simulink model "Aufgabe2_10"  (R2024b)
settings: Solver=ode4  StartTime=0.0  StopTime=200  FixedStep=0.01  RelTol=1e-3
values from neighbouring files (symbols this model uses):
  g = 9.807    [start.m]
undefined symbols (not defined in the file or in its folder): ft, INI, m, s
libraries: aerolibconvert2 x5, aerolibasang x4, slpidlib x3, aerolibanimutils x2, aerolibfltsims x2, simulink_extras x1, aerolibatmos2 x1, shared6dof x1
settings Model: Creator=annaf  LastModifiedBy=FrederikRittervonBae

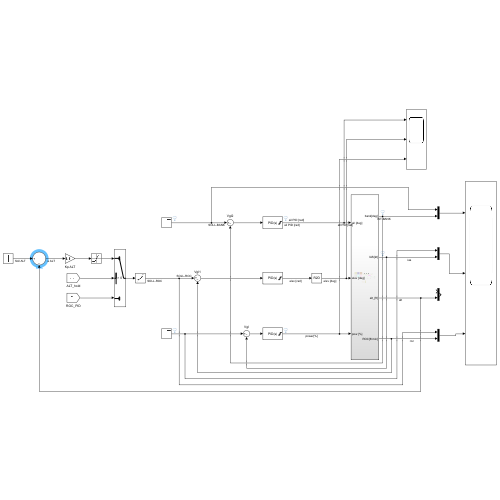
[thumbnail: Simulink's stored preview of the top-level diagram]
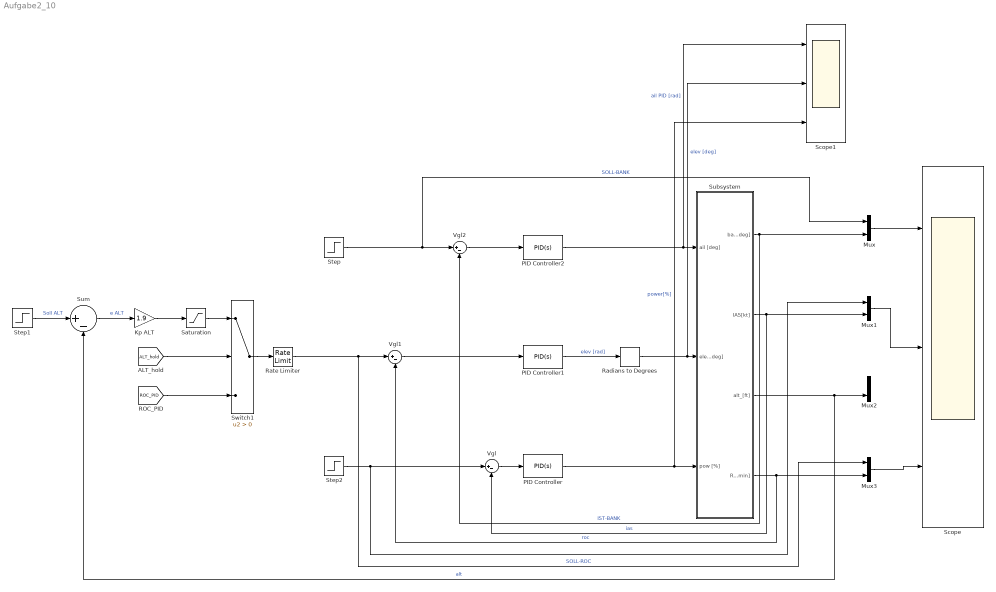
== system Aufgabe2_10 ==
  Kp ALT : Gain  Gain=1.9
  Mux{,1..3} (4 alike) : Mux  Inputs=2
  PID Controller : slpidlib/PID Controller  Controller=PID  Form=Parallel  TimeDomain=Continuous-time  UseExternalTs=off  SampleTime=-1  IntegratorMethod=Forward Euler  FilterMethod=Forward Euler  ControllerParametersSource=internal  P=68.6  I=5.4  UseKiTs=off  D=0.6  UseExternalDerivativeSource=off  N=100  UseFilter=on  TunerSelectOption=Transfer Function Based (PID Tuner App)  InitialConditionSource=internal  InitialConditionForIntegrator=0  InitialConditionForFilter=0  DifferentiatorICPrevScaledInput=0  ExternalReset=none  TrackingMode=off  Kt=1  LimitOutput=on  SatLimitsSource=internal  UpperSaturationLimit=100  LowerSaturationLimit=0  LinearizeAsGain=on  AntiWindupMode=clamping  Kb=1  LimitIntegrator=off  UpperIntegratorSaturationLimit=inf  LowerIntegratorSaturationLimit=-inf  POutMin=[]  POutMax=[]  IOutMin=[]  IOutMax=[]  DOutMin=[]  DOutMax=[]  NOutMin=[]  NOutMax=[]  SumOutMin=[]  SumOutMax=[]  SaturationOutMin=[]  SaturationOutMax=[]  PParamMin=[]  PParamMax=[]  IParamMin=[]  IParamMax=[]  DParamMin=[]  DParamMax=[]  NParamMin=[]  NParamMax=[]  KbParamMin=[]  KbParamMax=[]  KtParamMin=[]  KtParamMax=[]  KbOutMin=[]  KbOutMax=[]  KtOutMin=[]  KtOutMax=[]  IntegratorOutMin=[]  IntegratorOutMax=[]  FilterOutMin=[]  FilterOutMax=[]  SumI1OutMin=[]  SumI1OutMax=[]  SumI2OutMin=[]  SumI2OutMax=[]  SumI3OutMin=[]  SumI3OutMax=[]  SumI4OutMin=[]  SumI4OutMax=[]  SumDOutMin=[]  SumDOutMax=[]  DifferentiatorOutMin=[]  DifferentiatorOutMax=[]  FilterDiffOutCoefMin=[]  FilterDiffOutCoefMax=[]  ReciprocalOutMin=[]  ReciprocalOutMax=[]  SumDenOutMin=[]  SumDenOutMax=[]  SumNumOutMin=[]  SumNumOutMax=[]  DivideOutMin=[]  DivideOutMax=[]  UdiffTsProdOutMin=[]  UdiffTsProdOutMax=[]  NTsProdOutMin=[]  NTsProdOutMax=[]  UintegralTsProdOutMin=[]  UintegralTsProdOutMax=[]  UngainTsProdOutMin=[]  UngainTsProdOutMax=[]  ClampingZeroOutDataTypeStr=Inherit: Inherit via back propagation  ClampingZeroOutMin=[]  ClampingZeroOutMax=[]  FilterDenConstantOutDataTypeStr=Inherit: Inherit via back propagation  FilterDenConstantOutMin=[]  FilterDenConstantOutMax=[]  PCopyOutDataTypeStr=Inherit: Inherit via back propagation  PCopyOutMin=[]  PCopyOutMax=[]  NCopyOutDataTypeStr=Inherit: Inherit via back propagation  NCopyOutMin=[]  NCopyOutMax=[]  IntegratorContinuousStateAttributes=''  IntegratorStateMustResolveToSignalObject=off  IntegratorRTWStateStorageClass=Auto  FilterContinuousStateAttributes=''  FilterStateMustResolveToSignalObject=off  FilterRTWStateStorageClass=Auto  ParallelPVariant=InternalParameters  IdealPVariant=Disabled  IVariant=InternalParameters  DVariant=InternalParameters  IntegratorVariant=Continuous  SatVariant=Enabled  AWVariant=ContClampingParallel  PCopyVariant=Disabled  TRVariant=Disabled  FdbkBlocksVariant=Forward  IdealPFdbkVariant=Disabled  SatFdbkVariant=Disabled  DerivativeFilterVariant=ContFilter  NVariant=InternalParameters  NCopyVariant=Disabled  FilterICVariant=InternalICsFilter  IntegratorICVariant=InternalICs  ExternalResetVariant=Disabled  TRSumVariant=Passthrough  SumFdbkVariant=Disabled  SumVariant=Sum_PID  TsampFilterVariant=InternalTs  TsampNgainVariant=Passthrough  TsampIntegralVariant=Disabled_SignalSpec  ExternalSaturationOutDataTypeStr=Inherit: Same as second input  DerivativeSourceVariant=ErrorSignal  PreIntVariant=InternalPreInt
  PID Controller1 : slpidlib/PID Controller  Controller=PID  Form=Parallel  TimeDomain=Continuous-time  UseExternalTs=off  SampleTime=-1  IntegratorMethod=Forward Euler  FilterMethod=Forward Euler  ControllerParametersSource=internal  P=-0.14e-3  I=-0.032e-3  UseKiTs=off  D=-0.11e-3  UseExternalDerivativeSource=off  N=100  UseFilter=on  TunerSelectOption=Transfer Function Based (PID Tuner App)  InitialConditionSource=internal  InitialConditionForIntegrator=deg2rad(0.18948)  InitialConditionForFilter=0  DifferentiatorICPrevScaledInput=0  ExternalReset=none  TrackingMode=off  Kt=1  LimitOutput=on  SatLimitsSource=internal  UpperSaturationLimit=18 * pi/180  LowerSaturationLimit=-18 * pi/180  LinearizeAsGain=on  AntiWindupMode=clamping  Kb=1  LimitIntegrator=off  UpperIntegratorSaturationLimit=inf  LowerIntegratorSaturationLimit=-inf  POutMin=[]  POutMax=[]  IOutMin=[]  IOutMax=[]  DOutMin=[]  DOutMax=[]  NOutMin=[]  NOutMax=[]  SumOutMin=[]  SumOutMax=[]  SaturationOutMin=[]  SaturationOutMax=[]  PParamMin=[]  PParamMax=[]  IParamMin=[]  IParamMax=[]  DParamMin=[]  DParamMax=[]  NParamMin=[]  NParamMax=[]  KbParamMin=[]  KbParamMax=[]  KtParamMin=[]  KtParamMax=[]  KbOutMin=[]  KbOutMax=[]  KtOutMin=[]  KtOutMax=[]  IntegratorOutMin=[]  IntegratorOutMax=[]  FilterOutMin=[]  FilterOutMax=[]  SumI1OutMin=[]  SumI1OutMax=[]  SumI2OutMin=[]  SumI2OutMax=[]  SumI3OutMin=[]  SumI3OutMax=[]  SumI4OutMin=[]  SumI4OutMax=[]  SumDOutMin=[]  SumDOutMax=[]  DifferentiatorOutMin=[]  DifferentiatorOutMax=[]  FilterDiffOutCoefMin=[]  FilterDiffOutCoefMax=[]  ReciprocalOutMin=[]  ReciprocalOutMax=[]  SumDenOutMin=[]  SumDenOutMax=[]  SumNumOutMin=[]  SumNumOutMax=[]  DivideOutMin=[]  DivideOutMax=[]  UdiffTsProdOutMin=[]  UdiffTsProdOutMax=[]  NTsProdOutMin=[]  NTsProdOutMax=[]  UintegralTsProdOutMin=[]  UintegralTsProdOutMax=[]  UngainTsProdOutMin=[]  UngainTsProdOutMax=[]  ClampingZeroOutDataTypeStr=Inherit: Inherit via back propagation  ClampingZeroOutMin=[]  ClampingZeroOutMax=[]  FilterDenConstantOutDataTypeStr=Inherit: Inherit via back propagation  FilterDenConstantOutMin=[]  FilterDenConstantOutMax=[]  PCopyOutDataTypeStr=Inherit: Inherit via back propagation  PCopyOutMin=[]  PCopyOutMax=[]  NCopyOutDataTypeStr=Inherit: Inherit via back propagation  NCopyOutMin=[]  NCopyOutMax=[]  IntegratorContinuousStateAttributes=''  IntegratorStateMustResolveToSignalObject=off  IntegratorRTWStateStorageClass=Auto  FilterContinuousStateAttributes=''  FilterStateMustResolveToSignalObject=off  FilterRTWStateStorageClass=Auto  ParallelPVariant=InternalParameters  IdealPVariant=Disabled  IVariant=InternalParameters  DVariant=InternalParameters  IntegratorVariant=Continuous  SatVariant=Enabled  AWVariant=ContClampingParallel  PCopyVariant=Disabled  TRVariant=Disabled  FdbkBlocksVariant=Forward  IdealPFdbkVariant=Disabled  SatFdbkVariant=Disabled  DerivativeFilterVariant=ContFilter  NVariant=InternalParameters  NCopyVariant=Disabled  FilterICVariant=InternalICsFilter  IntegratorICVariant=InternalICs  ExternalResetVariant=Disabled  TRSumVariant=Passthrough  SumFdbkVariant=Disabled  SumVariant=Sum_PID  TsampFilterVariant=InternalTs  TsampNgainVariant=Passthrough  TsampIntegralVariant=Disabled_SignalSpec  ExternalSaturationOutDataTypeStr=Inherit: Same as second input  DerivativeSourceVariant=ErrorSignal  PreIntVariant=InternalPreInt
  PID Controller2 : slpidlib/PID Controller  Controller=PID  Form=Parallel  TimeDomain=Continuous-time  UseExternalTs=off  SampleTime=-1  IntegratorMethod=Forward Euler  FilterMethod=Forward Euler  ControllerParametersSource=internal  P=-2.30711584231478  I=-1.20407962427496  UseKiTs=off  D=-0.00333321729170639  UseExternalDerivativeSource=off  N=5.47913427920366  UseFilter=on  TunerSelectOption=Transfer Function Based (PID Tuner App)  InitialConditionSource=internal  InitialConditionForIntegrator=0  InitialConditionForFilter=0  DifferentiatorICPrevScaledInput=0  ExternalReset=none  TrackingMode=off  Kt=1  LimitOutput=on  SatLimitsSource=internal  UpperSaturationLimit=20  LowerSaturationLimit=-20  LinearizeAsGain=on  AntiWindupMode=clamping  Kb=1  LimitIntegrator=off  UpperIntegratorSaturationLimit=inf  LowerIntegratorSaturationLimit=-inf  POutMin=[]  POutMax=[]  IOutMin=[]  IOutMax=[]  DOutMin=[]  DOutMax=[]  NOutMin=[]  NOutMax=[]  SumOutMin=[]  SumOutMax=[]  SaturationOutMin=[]  SaturationOutMax=[]  PParamMin=[]  PParamMax=[]  IParamMin=[]  IParamMax=[]  DParamMin=[]  DParamMax=[]  NParamMin=[]  NParamMax=[]  KbParamMin=[]  KbParamMax=[]  KtParamMin=[]  KtParamMax=[]  KbOutMin=[]  KbOutMax=[]  KtOutMin=[]  KtOutMax=[]  IntegratorOutMin=[]  IntegratorOutMax=[]  FilterOutMin=[]  FilterOutMax=[]  SumI1OutMin=[]  SumI1OutMax=[]  SumI2OutMin=[]  SumI2OutMax=[]  SumI3OutMin=[]  SumI3OutMax=[]  SumI4OutMin=[]  SumI4OutMax=[]  SumDOutMin=[]  SumDOutMax=[]  DifferentiatorOutMin=[]  DifferentiatorOutMax=[]  FilterDiffOutCoefMin=[]  FilterDiffOutCoefMax=[]  ReciprocalOutMin=[]  ReciprocalOutMax=[]  SumDenOutMin=[]  SumDenOutMax=[]  SumNumOutMin=[]  SumNumOutMax=[]  DivideOutMin=[]  DivideOutMax=[]  UdiffTsProdOutMin=[]  UdiffTsProdOutMax=[]  NTsProdOutMin=[]  NTsProdOutMax=[]  UintegralTsProdOutMin=[]  UintegralTsProdOutMax=[]  UngainTsProdOutMin=[]  UngainTsProdOutMax=[]  ClampingZeroOutDataTypeStr=Inherit: Inherit via back propagation  ClampingZeroOutMin=[]  ClampingZeroOutMax=[]  FilterDenConstantOutDataTypeStr=Inherit: Inherit via back propagation  FilterDenConstantOutMin=[]  FilterDenConstantOutMax=[]  PCopyOutDataTypeStr=Inherit: Inherit via back propagation  PCopyOutMin=[]  PCopyOutMax=[]  NCopyOutDataTypeStr=Inherit: Inherit via back propagation  NCopyOutMin=[]  NCopyOutMax=[]  IntegratorContinuousStateAttributes=''  IntegratorStateMustResolveToSignalObject=off  IntegratorRTWStateStorageClass=Auto  FilterContinuousStateAttributes=''  FilterStateMustResolveToSignalObject=off  FilterRTWStateStorageClass=Auto  ParallelPVariant=InternalParameters  IdealPVariant=Disabled  IVariant=InternalParameters  DVariant=InternalParameters  IntegratorVariant=Continuous  SatVariant=Enabled  AWVariant=ContClampingParallel  PCopyVariant=Disabled  TRVariant=Disabled  FdbkBlocksVariant=Forward  IdealPFdbkVariant=Disabled  SatFdbkVariant=Disabled  DerivativeFilterVariant=ContFilter  NVariant=InternalParameters  NCopyVariant=Disabled  FilterICVariant=InternalICsFilter  IntegratorICVariant=InternalICs  ExternalResetVariant=Disabled  TRSumVariant=Passthrough  SumFdbkVariant=Disabled  SumVariant=Sum_PID  TsampFilterVariant=InternalTs  TsampNgainVariant=Passthrough  TsampIntegralVariant=Disabled_SignalSpec  ExternalSaturationOutDataTypeStr=Inherit: Same as second input  DerivativeSourceVariant=ErrorSignal  PreIntVariant=InternalPreInt
  Radians to Degrees : simulink_extras/Transformations/Radians to Degrees
  Rate Limiter : RateLimiter  RisingSlewLimit=70  FallingSlewLimit=-70  SampleTimeMode=inherited
  Saturation : Saturate  UpperLimit=1200  LowerLimit=-1200
  Scope : Scope  NumInputPorts=3
  Scope1 : Scope  NumInputPorts=3
  Step : Step  Time=60  After=0  SampleTime=0
  Step1 : Step  Time=30  Before=1000  After=1200  SampleTime=0
  Step2 : Step  Before=60  After=60  SampleTime=0
  Subsystem : Subsystem
  Sum : Sum  Inputs=|+-
  Switch1 : Switch  Criteria=u2 > Threshold  SaturateOnIntegerOverflow=off  InputSameDT=off
  Vgl : Sum  Inputs=|+-
  Vgl1 : Sum  Inputs=|+-
  Vgl2 : Sum  Inputs=|+-
  wires:
  Subsystem/1(bank[deg]) -> Mux/2, Vgl2/2  "IST-BANK"
  Subsystem/3(alt_[ft]) -> Sum/2, Mux2/2  "alt"
  Subsystem/4(ROC[ft/min]) -> Mux3/2, Vgl1/2  "roc"
  PID Controller/1 -> Scope1/3, Subsystem/3(pow [%])  "power[%]"
  Step2/1 -> Vgl/1, Mux1/1
  Subsystem/2(IAS[kt]) -> Mux1/2, Vgl/2  "ias"
  Vgl/1 -> PID Controller/1
  Kp ALT/1 -> Saturation/1
  [ROC_PID] -> Switch1/3
  Saturation/1 -> Switch1/1
  PID Controller1/1 -> Radians to Degrees/1  "elev [rad]"
  Vgl1/1 -> PID Controller1/1
  Sum/1 -> Kp ALT/1  "e ALT"
  Switch1/1 -> Rate Limiter/1
  Radians to Degrees/1 -> Scope1/2, Subsystem/2(elev [deg])  "elev [deg]"
  [ALT_hold] -> Switch1/2
  Step/1 -> Vgl2/1, Mux/1  "SOLL-BANK"
  PID Controller2/1 -> Scope1/1, Subsystem/1(ail [deg])  "ail PID [rad]"
  Step1/1 -> Sum/1  "Soll ALT"
  Mux/1 -> Scope/1
  Mux1/1 -> Scope/2
  Mux3/1 -> Scope/3
  Vgl2/1 -> PID Controller2/1
  Rate Limiter/1 -> Mux3/1, Vgl1/1  "SOLL-ROC"

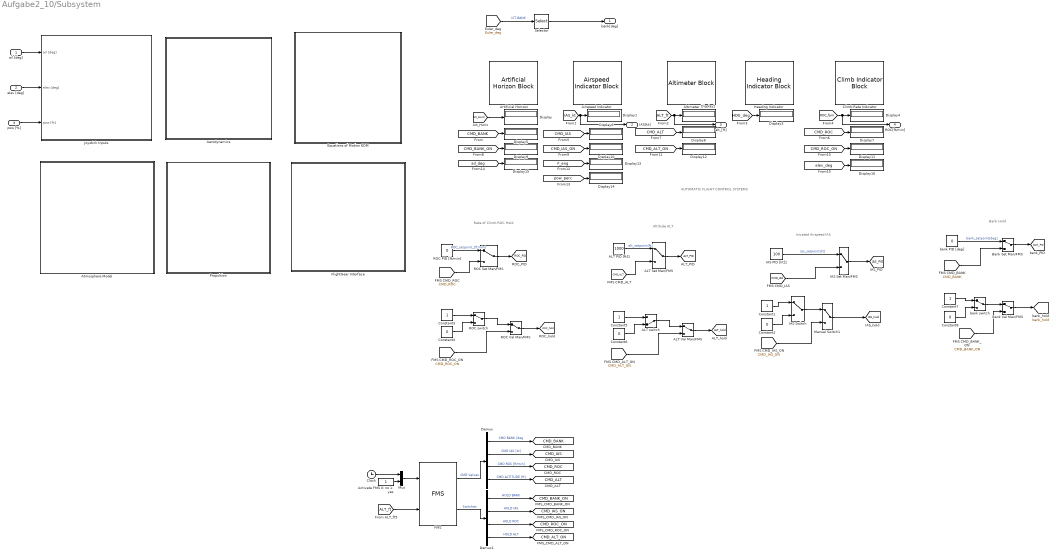
== system Aufgabe2_10/Subsystem ==
  note: AUTOMATIC FLIGHT CONTROL SYSTEMS
  note: Altitude ALT
  note: Rate of Climb ROC Hold
  note: Bank Hold
  note: Inicated Airspeed IAS
  ail [deg] : Inport
  elev [deg] : Inport  Port=2
  pow [%] : Inport  Port=3
  " bank switch" : ManualSwitch
  ALT PID [ft]1 : Constant  Value=1000
  ALT Set Man/FMS : ManualSwitch
  ALT Val Man/FMS : ManualSwitch
  ALT switch : ManualSwitch  CurrentSetting=0
  Activate FMS 0: no 1: yes : Constant
  Aerodynamics : Subsystem
  Airspeed Indicator : AirspeedIndicatorBlock
  Altimeter : AltimeterBlock
  Artificial Horizon : ArtificialHorizonBlock
  Atmosphere Model : Subsystem
  Bank Set Man/FMS : ManualSwitch
  Bank Val Man/FMS : ManualSwitch
  Climb Rate Indicator : ClimbIndicatorBlock
  Clock : Clock
  Constant{1,3,5,7} (4 alike) : Constant
  Constant{2,4,6,8} (4 alike) : Constant  Value=0
  Demux : Demux
  Demux1 : Demux
  Display{,1..16} (17 alike) : Display
  Equations of Motion EOM : Subsystem
  FMS : M-S-Function  FunctionName=FMS
  FlightGear Interface : Subsystem
  Heading Indicator : HeadingIndicatorBlock
  IAS PID [kt]1 : Constant  Value=100
  IAS Set Man/FMS : ManualSwitch
  IAS Switch : ManualSwitch
  Joystick Inputs : Subsystem
  Manual Switch1 : ManualSwitch
  Mux : Mux  Inputs=2
  Propulsion : Subsystem
  ROC PID [ft/min] : Constant  Value=0
  ROC Set Man/FMS : ManualSwitch
  ROC Val Man/FMS : ManualSwitch
  ROC switch : ManualSwitch
  Selector : Selector  InputPortWidth=3  IndexOptions=Index vector (dialog)  Indices=1  OutputSizes=1
  bank PID [deg] : Constant  Value=0
  bank[deg] : Outport
  IAS[kt] : Outport  Port=2
  alt_[ft] : Outport  Port=3
  ROC[ft/min] : Outport  Port=4
  tag scope: ALT_PID=global, ALT_hold=global, CMD_ALT=global, CMD_ALT_ON=global, CMD_BANK=global, CMD_BANK_ON=global, CMD_IAS=global, CMD_IAS_ON=global, CMD_ROC=global, CMD_ROC_ON=global, IAS_PID=global, IAS_hold=global, ROC_PID=global, ROC_hold=global, bank_PID=global, bank_hold=global
  wires:
  [CMD_IAS_ON] -> Manual Switch1/2
  ALT Val Man/FMS/1 -> [ALT_hold]
  [ALT_ft] -> alt_[ft]/1, Display2/1
  [CMD_IAS] -> Display6/1
  Constant4/1 -> ROC switch/2
  Demux/2 -> [CMD_IAS]  "CMD IAS [kt]"
  Bank Val Man/FMS/1 -> [bank_hold]
  Demux/4 -> [CMD_ALT]  "CMD ALTITUDE [ft]"
  ROC Set Man/FMS/1 -> [ROC_PID]
  " bank switch"/1 -> Bank Val Man/FMS/1
  [CMD_IAS_ON] -> Display10/1
  ALT PID [ft]1/1 -> ALT Set Man/FMS/1  "alt_setpoint[ft]"
  ROC switch/1 -> ROC Val Man/FMS/1
  [CMD_BANK_ON] -> Display9/1
  [CMD_ROC] -> ROC Set Man/FMS/2
  [F_eng] -> Display13/1
  [ail_deg] -> Display15/1
  [CMD_ROC_ON] -> ROC Val Man/FMS/2
  Constant2/1 -> IAS Switch/2
  [CMD_ROC_ON] -> Display11/1
  ALT switch/1 -> ALT Val Man/FMS/1
  Constant7/1 -> " bank switch"/1
  [IAS_kt] -> IAS[kt]/1, Display1/1
  [CMD_ALT_ON] -> ALT Val Man/FMS/2
  [CMD_BANK_ON] -> Bank Val Man/FMS/2
  FMS/2 -> Demux1/1  "Switches"
  Constant3/1 -> ROC switch/1
  [HDG_deg] -> Display3/1
  bank PID [deg]/1 -> Bank Set Man/FMS/1  "bank_setpoint[deg]"
  Activate FMS 0: no 1: yes/1 -> Mux/2
  [CMD_IAS] -> IAS Set Man/FMS/2
  Constant5/1 -> ALT switch/1
  [pow_perc] -> Display14/1
  Demux1/1 -> [CMD_BANK_ON]  "HOLD BANK"
  Manual Switch1/1 -> [IAS_hold]
  [CMD_ALT] -> ALT Set Man/FMS/2
  Constant1/1 -> IAS Switch/1
  Demux/1 -> [CMD_BANK]  "CMD BANK [deg"
  Constant8/1 -> " bank switch"/2
  [CMD_ALT] -> Display8/1
  [ALT_ft] -> FMS/2
  [ROC_fpm] -> ROC[ft/min]/1, Display4/1
  [CMD_ALT_ON] -> Display12/1
  Bank Set Man/FMS/1 -> [bank_PID]
  ALT Set Man/FMS/1 -> [ALT_PID]
  Demux1/2 -> [CMD_IAS_ON]  "HOLD IAS"
  IAS PID [kt]1/1 -> IAS Set Man/FMS/1  "ias_setpoint[kt]"
  Demux1/3 -> [CMD_ROC_ON]  "HOLD ROC"
  Demux/3 -> [CMD_ROC]  "CMD ROC [ft/min]"
  [elev_deg] -> Display16/1
  ROC PID [ft/min]/1 -> ROC Set Man/FMS/1  "ROC_setpoint_[ft/min]"
  [CMD_BANK] -> Bank Set Man/FMS/2
  ROC Val Man/FMS/1 -> [ROC_hold]
  [Art_Horiz] -> Display/1
  Mux/1 -> FMS/1
  Demux1/4 -> [CMD_ALT_ON]  "HOLD ALT"
  Clock/1 -> Mux/1
  FMS/1 -> Demux/1  "CMD Values"
  Constant6/1 -> ALT switch/2
  IAS Switch/1 -> Manual Switch1/1
  [CMD_ROC] -> Display7/1
  IAS Set Man/FMS/1 -> [IAS_PID]
  ail [deg]/1 -> Joystick Inputs/1(ail [deg])
  elev [deg]/1 -> Joystick Inputs/2(elev [deg])
  pow [%]/1 -> Joystick Inputs/3(pow [%])
  [CMD_BANK] -> Display5/1
  Selector/1 -> bank[deg]/1
  [Euler_deg] -> Selector/1  "IST-BANK"

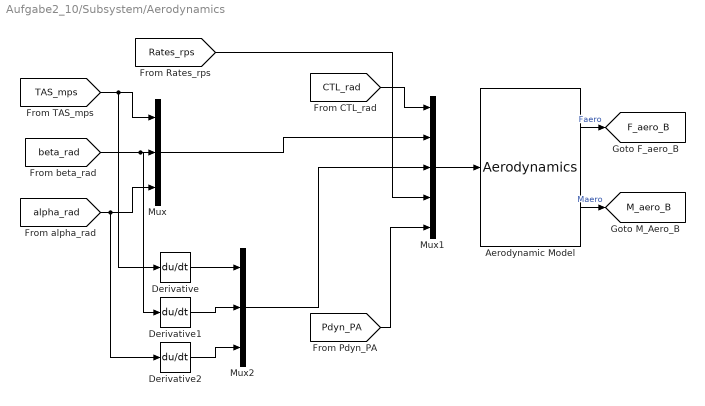
== system Aufgabe2_10/Subsystem/Aerodynamics ==
  Aerodynamic Model : M-S-Function  FunctionName=Aerodynamics
  Derivative : Derivative
  Derivative1 : Derivative
  Derivative2 : Derivative
  Mux : Mux  Inputs=3
  Mux1 : Mux  Inputs=5
  Mux2 : Mux  Inputs=3
  tag scope: F_aero_B=global, M_aero_B=global
  wires:
  [beta_rad] -> Derivative1/1, Mux/2
  Aerodynamic Model/2 -> [M_aero_B]  "Maero"
  [TAS_mps] -> Derivative/1, Mux/1
  [Pdyn_PA] -> Mux1/5
  [CTL_rad] -> Mux1/1
  Aerodynamic Model/1 -> [F_aero_B]  "Faero"
  [alpha_rad] -> Derivative2/1, Mux/3
  Mux1/1 -> Aerodynamic Model/1
  Mux/1 -> Mux1/2
  [Rates_rps] -> Mux1/4
  Derivative/1 -> Mux2/1
  Derivative1/1 -> Mux2/2
  Derivative2/1 -> Mux2/3
  Mux2/1 -> Mux1/3

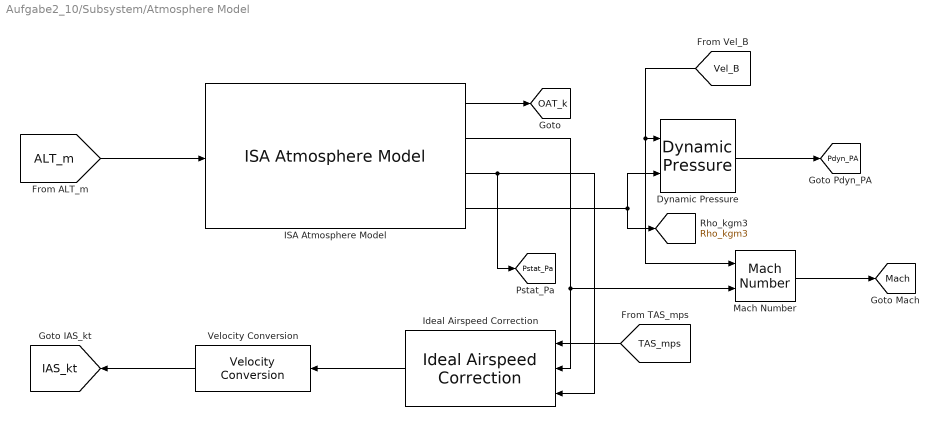
== system Aufgabe2_10/Subsystem/Atmosphere Model ==
  Dynamic Pressure : aerolibasang/Dynamic Pressure
  ISA Atmosphere Model : aerolibatmos2/ISA Atmosphere Model  useExtended=off  action=Warning  custom=off  viscosityOut=off  g=9.80665  gamma=1.4  R=287.0531  L=0.0065  h_trop=11000  h_strat=20000  rho0=1.225  P0=101325  T0=288.15  h0=0  S=110.4  Tref=273.15  muref=1.716e-5
  Ideal Airspeed Correction : aerolibasang/Ideal Airspeed Correction  units=Metric (MKS)  vel_in=TAS  vel_out_tas=EAS  vel_out_eas=TAS  vel_out_cas=TAS  method=Table Lookup  SubOnly=off  action=None
  Mach Number : aerolibasang/Mach Number
  Velocity Conversion : aerolibconvert2/Velocity Conversion  IU=m/s  OU=kts
  tag scope: IAS_kt=global, Mach=global, OAT_k=global, Pdyn_PA=global, Pstat_Pa=global, Rho_kgm3=global
  wires:
  Velocity Conversion/1 -> [IAS_kt]
  ISA Atmosphere Model/1 -> [OAT_k]
  ISA Atmosphere Model/4 -> [Rho_kgm3], Dynamic Pressure/2
  [Vel_B] -> Mach Number/1, Dynamic Pressure/1
  [ALT_m] -> ISA Atmosphere Model/1
  Mach Number/1 -> [Mach]
  Dynamic Pressure/1 -> [Pdyn_PA]
  ISA Atmosphere Model/3 -> [Pstat_Pa], Ideal Airspeed Correction/3
  [TAS_mps] -> Ideal Airspeed Correction/1
  ISA Atmosphere Model/2 -> Mach Number/2, Ideal Airspeed Correction/2
  Ideal Airspeed Correction/1 -> Velocity Conversion/1

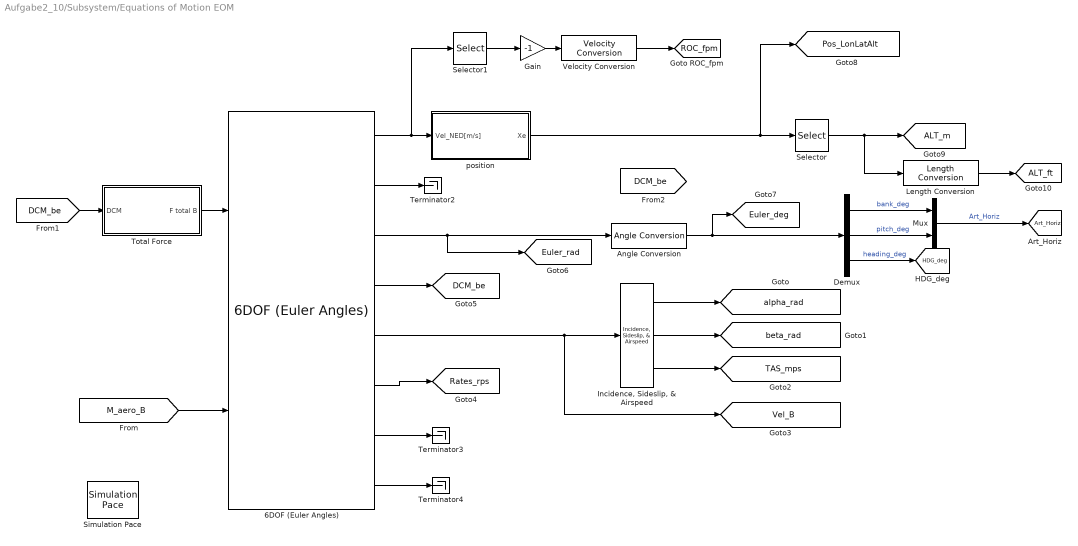
== system Aufgabe2_10/Subsystem/Equations of Motion EOM ==
  6DOF (Euler Angles) : shared6dof/6DOF (Euler Angles)  units=Metric (MKS)  mtype=Fixed  rep=Euler Angles  xme_0=INI.POS'  Vm_0=INI.VELbod'  eul_0=INI.EULER'  pm_0=INI.PQR'  mass_0=INI.mass  mass_e=0.5  mass_f=2.0  inertia=INI.Inertia  inertia_e=eye(3)  inertia_f=2*eye(3)  k_quat=1.0  vre_flag=on  abi_flag=off  aMode=0  xme_statename=''  Vm_statename=''  eul_statename=''  quat_statename=''  pm_statename=''  mass_statename=''
  Angle Conversion : aerolibconvert2/Angle Conversion  IU=rad  OU=deg
  Demux : Demux  Outputs=3
  Gain : Gain  Gain=-1
  "Incidence, Sideslip, & Airspeed" : aerolibasang/Incidence, Sideslip, & Airspeed
  Length Conversion : aerolibconvert2/Length Conversion  IU=m  OU=ft
  Mux : Mux  Inputs=2
  Selector : Selector  InputPortWidth=3  IndexOptions=Starting index (dialog)  Indices=3  OutputSizes=1
  Selector1 : Selector  InputPortWidth=3  IndexOptions=Starting index (dialog)  Indices=3  OutputSizes=1
  Simulation Pace : aerolibanimutils/Simulation Pace  SimulationPace=1  SleepMode=Auto  OutputPaceError=off  SampleTime=sampletime
  Terminator2 : Terminator
  Terminator3 : Terminator
  Terminator4 : Terminator
  Total Force : Subsystem
  Velocity Conversion : aerolibconvert2/Velocity Conversion  IU=m/s  OU=ft/min
  position : Subsystem
  tag scope: ALT_ft=global, ALT_m=global, Art_Horiz=global, DCM_be=global, Euler_deg=global, Euler_rad=global, HDG_deg=global, Pos_LonLatAlt=global, ROC_fpm=global, Rates_rps=global, TAS_mps=global, Vel_B=global, alpha_rad=global, beta_rad=global
  wires:
  6DOF (Euler Angles)/5 -> [Vel_B], "Incidence, Sideslip, & Airspeed"/1
  "Incidence, Sideslip, & Airspeed"/1 -> [alpha_rad]
  "Incidence, Sideslip, & Airspeed"/2 -> [beta_rad]
  "Incidence, Sideslip, & Airspeed"/3 -> [TAS_mps]
  6DOF (Euler Angles)/6 -> [Rates_rps]
  [M_aero_B] -> 6DOF (Euler Angles)/2
  Total Force/1(F total B) -> 6DOF (Euler Angles)/1
  [DCM_be] -> Total Force/1(DCM)
  6DOF (Euler Angles)/4 -> [DCM_be]
  6DOF (Euler Angles)/3 -> Angle Conversion/1, [Euler_rad]
  Angle Conversion/1 -> Demux/1, [Euler_deg]
  Demux/1 -> Mux/1  "bank_deg"
  Demux/2 -> Mux/2  "pitch_deg"
  Mux/1 -> [Art_Horiz]  "Art_Horiz"
  Demux/3 -> [HDG_deg]  "heading_deg"
  6DOF (Euler Angles)/2 -> Terminator2/1
  position/1(Xe) -> [Pos_LonLatAlt], Selector/1
  Selector/1 -> Length Conversion/1, [ALT_m]
  Length Conversion/1 -> [ALT_ft]
  6DOF (Euler Angles)/7 -> Terminator3/1
  6DOF (Euler Angles)/8 -> Terminator4/1
  Velocity Conversion/1 -> [ROC_fpm]
  Selector1/1 -> Gain/1
  6DOF (Euler Angles)/1 -> Selector1/1, position/1(Vel_NED[m/s])
  Gain/1 -> Velocity Conversion/1

== system Aufgabe2_10/Subsystem/FlightGear Interface ==
  Cast To Single : DataTypeConversion  OutDataTypeStr=single  SaturateOnIntegerOverflow=off  RndMeth=Floor
  Demux : Demux  Outputs=3
  Demux1 : Demux  Outputs=3
  Pack net_fdm Packet for FlightGear : aerolibfltsims/Pack net_fdm Packet for FlightGear  FlightGearVersion=v2019.1  ShowPositionAttitudeInputs=on  ShowVelocityAccelerationInputs=off  ShowControlSurfacePositionInputs=off  ShowEngineFuelInputs=off  ShowLandingGearInputs=off  ShowEnvironmentInputs=off  SampleTime=sampletime  packetVersion=24
  Scope : Scope  NumInputPorts=6
  Send net_fdm Packet to FlightGear : aerolibfltsims/Send net_fdm Packet to FlightGear  DestinationIpAddress=127.0.0.1  DestinationPort=5502  LocalIpPort=-1  varLen=off  SampleTime=sampletime
  wires:
  Pack net_fdm Packet for FlightGear/1 -> Send net_fdm Packet to FlightGear/1
  [Pos_LonLatAlt] -> Demux/1
  Demux/1 -> Pack net_fdm Packet for FlightGear/1, Scope/1  "l"
  Demux/2 -> Scope/2, Pack net_fdm Packet for FlightGear/2  "mü"
  Demux/3 -> Scope/3, Pack net_fdm Packet for FlightGear/3  "h"
  [Euler_rad] -> Cast To Single/1
  Cast To Single/1 -> Demux1/1
  Demux1/1 -> Scope/4, Pack net_fdm Packet for FlightGear/4  "Rollw"
  Demux1/2 -> Scope/5, Pack net_fdm Packet for FlightGear/5  "Nickw"
  Demux1/3 -> Scope/6, Pack net_fdm Packet for FlightGear/6  "Gierw"

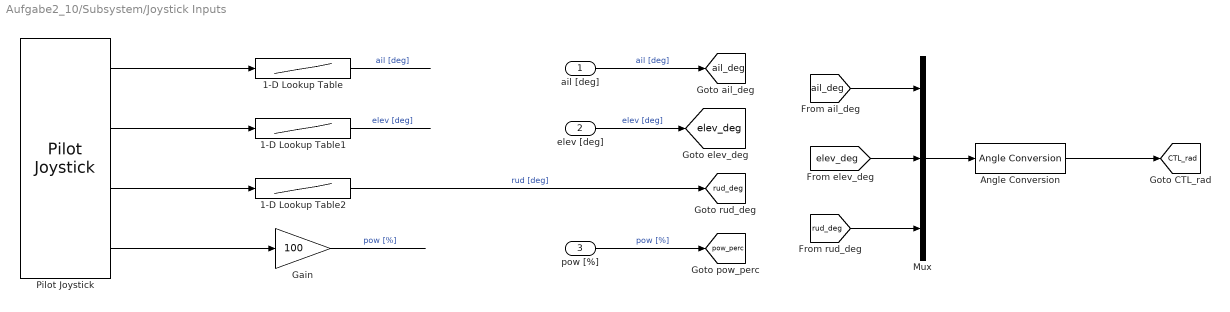
== system Aufgabe2_10/Subsystem/Joystick Inputs ==
  ail [deg] : Inport
  elev [deg] : Inport  Port=2
  pow [%] : Inport  Port=3
  1-D Lookup Table : Lookup_n-D  NumberOfTableDimensions=1  BreakpointsForDimension1=[-1 0 1]  Table=[20 0 -20]  InternalRulePriority=Speed  RndMeth=Simplest
  1-D Lookup Table1 : Lookup_n-D  NumberOfTableDimensions=1  BreakpointsForDimension1=[-1 0 1]  Table=[18 0 -18]  InternalRulePriority=Speed  RndMeth=Simplest
  1-D Lookup Table2 : Lookup_n-D  NumberOfTableDimensions=1  BreakpointsForDimension1=[-1 0 1]  Table=[-25 0 25]  InternalRulePriority=Speed  RndMeth=Simplest
  Angle Conversion : aerolibconvert2/Angle Conversion  IU=deg  OU=rad
  Gain : Gain  Gain=100
  Mux : Mux  Inputs=3
  Pilot Joystick : aerolibanimutils/Pilot Joystick  JoystickID=None  OutputConfiguration=FourAxis  SampleTime=sampletime
  tag scope: CTL_rad=global, ail_deg=global, elev_deg=global, pow_perc=global, rud_deg=global
  wires:
  Angle Conversion/1 -> [CTL_rad]
  [elev_deg] -> Mux/2
  [rud_deg] -> Mux/3
  Mux/1 -> Angle Conversion/1
  1-D Lookup Table2/1 -> [rud_deg]  "rud [deg]"
  1-D Lookup Table1/1 -> ?  "elev [deg]"
  1-D Lookup Table/1 -> ?  "ail [deg]"
  Gain/1 -> ?  "pow [%]"
  [ail_deg] -> Mux/1
  Pilot Joystick/2 -> 1-D Lookup Table1/1
  Pilot Joystick/3 -> 1-D Lookup Table2/1
  Pilot Joystick/4 -> Gain/1
  Pilot Joystick/1 -> 1-D Lookup Table/1
  pow [%]/1 -> [pow_perc]  "pow [%]"
  elev [deg]/1 -> [elev_deg]  "elev [deg]"
  ail [deg]/1 -> [ail_deg]  "ail [deg]"

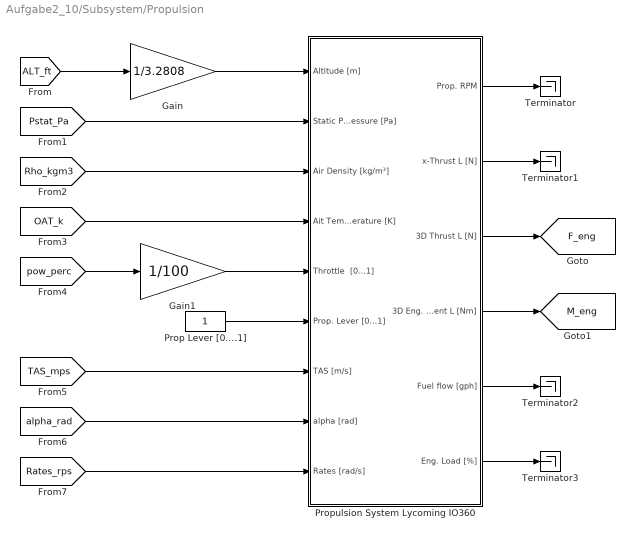
== system Aufgabe2_10/Subsystem/Propulsion ==
  Gain : Gain  Gain=1/3.2808
  Gain1 : Gain  Gain=1/100
  Prop Lever [0....1] : Constant
  Propulsion System Lycoming IO360 : Subsystem  mask{Y_TW=0}
      mask prompts: Y_TW "Y Position of the Engine [m]. Positive for Left Engine"
  Terminator{,1..3} (4 alike) : Terminator
  tag scope: F_eng=global, M_eng=global
  wires:
  [ALT_ft] -> Gain/1
  [pow_perc] -> Gain1/1
  Propulsion System Lycoming IO360/6(Eng. Load [%]) -> Terminator3/1
  [alpha_rad] -> Propulsion System Lycoming IO360/8(alpha [rad])
  Propulsion System Lycoming IO360/1(Prop. RPM) -> Terminator/1
  [TAS_mps] -> Propulsion System Lycoming IO360/7(TAS [m/s])
  [Pstat_Pa] -> Propulsion System Lycoming IO360/2(Static Pressure [Pa])
  Propulsion System Lycoming IO360/3(3D Thrust L [N]) -> [F_eng]
  Propulsion System Lycoming IO360/4(3D Eng. Moment L [Nm]) -> [M_eng]
  Propulsion System Lycoming IO360/2(x-Thrust L [N]) -> Terminator1/1
  Gain1/1 -> Propulsion System Lycoming IO360/5(Throttle  [0...1])
  Prop Lever [0....1]/1 -> Propulsion System Lycoming IO360/6(Prop. Lever [0...1])
  [Rates_rps] -> Propulsion System Lycoming IO360/9(Rates [rad/s])
  Gain/1 -> Propulsion System Lycoming IO360/1(Altitude [m])
  Propulsion System Lycoming IO360/5(Fuel flow [gph]) -> Terminator2/1
  [OAT_k] -> Propulsion System Lycoming IO360/4(Ait Temperature [K])
  [Rho_kgm3] -> Propulsion System Lycoming IO360/3(Air Density [kg/m³])

== system Aufgabe2_10/Subsystem/Equations of Motion EOM/Total Force ==
  DCM : Inport
  Add : Sum
  Add2 : Sum
  Gravity [m/s²] : Constant  Value=[0 0 g]
  Product : Product
  Product1 : Product  Multiplication=Matrix(*)
  aircraft mass [kg] : Constant  Value=INI.mass
  F total B : Outport  VectorParamsAs1DForOutWhenUnconnected=off
  wires:
  Add/1 -> Add2/1
  Gravity [m/s²]/1 -> Product/2
  Product1/1 -> Add2/2
  Add2/1 -> F total B/1
  Product/1 -> Product1/2
  aircraft mass [kg]/1 -> Product/1
  DCM/1 -> Product1/1
  [F_eng] -> Add/2
  [F_aero_B] -> Add/1

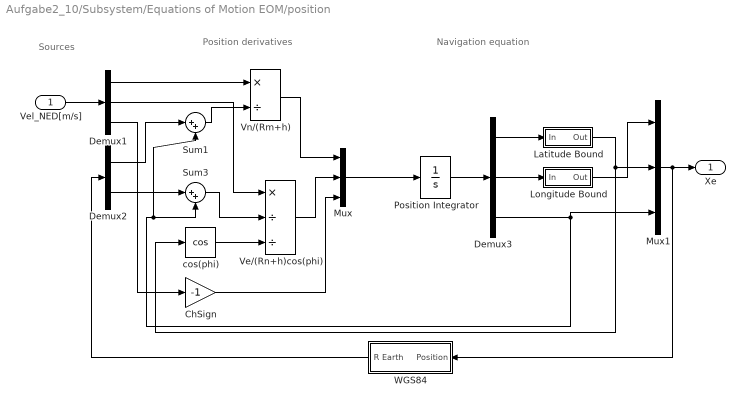
== system Aufgabe2_10/Subsystem/Equations of Motion EOM/position ==
  note: Navigation equation
  note: Position derivatives
  note: Sources
  Vel_NED[m/s] : Inport
  ChSign : Gain  Gain=-1  SaturateOnIntegerOverflow=on  OutDataTypeStr=Inherit: Same as input  ParamDataTypeStr=Inherit: Same as input
  Demux1 : Demux  Outputs=3
      settings: DisplayOption=none
  Demux2 : Demux  Outputs=2
      settings: DisplayOption=none
  Demux3 : Demux  Outputs=3
      settings: DisplayOption=none
  Latitude Bound : Subsystem
  Longitude Bound : Subsystem
  Mux : Mux  Inputs=3
  Mux1 : Mux  Inputs=3
  Position Integrator : Integrator  InitialCondition=INI.POS
  Sum1 : Sum  Inputs=|++
  Sum3 : Sum  Inputs=|++
  Ve/(Rn+h)cos(phi) : Product  Inputs=*//  InputSameDT=on  SaturateOnIntegerOverflow=on  OutDataTypeStr=Inherit: Same as first input
  Vn/(Rm+h) : Product  Inputs=*/  InputSameDT=on  SaturateOnIntegerOverflow=on  OutDataTypeStr=Inherit: Same as first input
  WGS84 : Subsystem
  cos(phi) : Trigonometry  Operator=cos
  Xe : Outport  VectorParamsAs1DForOutWhenUnconnected=off
  wires:
  Longitude Bound/1(Out) -> Mux1/1
  Mux1/1 -> Xe/1, WGS84/1(Position)
  cos(phi)/1 -> Ve/(Rn+h)cos(phi)/3
  Demux3/1 -> Latitude Bound/1(In)
  ChSign/1 -> Mux/3
  Latitude Bound/1(Out) -> cos(phi)/1, Mux1/2
  Vn/(Rm+h)/1 -> Mux/1
  Demux1/2 -> Ve/(Rn+h)cos(phi)/1
  Demux1/1 -> Vn/(Rm+h)/1
  Vel_NED[m/s]/1 -> Demux1/1
  Demux1/3 -> ChSign/1
  Demux3/2 -> Longitude Bound/1(In)
  Demux3/3 -> Mux1/3, Sum3/2, Sum1/2
  Ve/(Rn+h)cos(phi)/1 -> Mux/2
  WGS84/1(R Earth) -> Demux2/1
  Sum1/1 -> Vn/(Rm+h)/2
  Demux2/1 -> Sum1/1
  Demux2/2 -> Sum3/1
  Sum3/1 -> Ve/(Rn+h)cos(phi)/2
  Position Integrator/1 -> Demux3/1
  Mux/1 -> Position Integrator/1

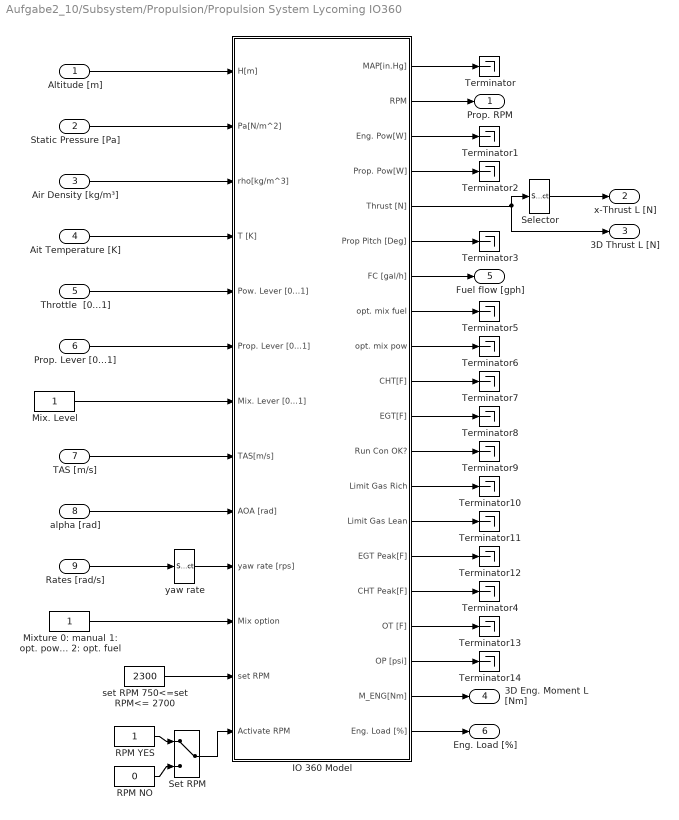
== system Aufgabe2_10/Subsystem/Propulsion/Propulsion System Lycoming IO360 ==
  Altitude [m] : Inport
  Static Pressure [Pa] : Inport  Port=2
  Air Density [kg/m³] : Inport  Port=3
  Ait Temperature [K] : Inport  Port=4
  Throttle  [0...1] : Inport  Port=5
  Prop. Lever [0...1] : Inport  Port=6
  TAS [m/s] : Inport  Port=7
  alpha [rad] : Inport  Port=8
  Rates [rad/s] : Inport  Port=9
  IO 360 Model : Subsystem
  "Mix. Level " : Constant
  "Mixture 0: manual 1: opt. pow 2: opt. fuel " : Constant
  RPM NO : Constant  Value=0
  RPM YES : Constant
  Selector : Selector  InputPortWidth=3  IndexOptions=Index vector (dialog)  Indices=1  OutputSizes=1
  Set RPM : ManualSwitch
  Terminator{,1..14} (15 alike) : Terminator
  set RPM 750<=set RPM<= 2700 : Constant  Value=2300
  yaw rate : Selector  InputPortWidth=3  IndexOptions=Index vector (dialog)  Indices=3  OutputSizes=1
  Prop. RPM : Outport  VectorParamsAs1DForOutWhenUnconnected=off
  x-Thrust L [N] : Outport  Port=2  VectorParamsAs1DForOutWhenUnconnected=off
  3D Thrust L [N] : Outport  Port=3  VectorParamsAs1DForOutWhenUnconnected=off
  3D Eng. Moment L [Nm] : Outport  Port=4  VectorParamsAs1DForOutWhenUnconnected=off
  Fuel flow [gph] : Outport  Port=5  VectorParamsAs1DForOutWhenUnconnected=off
  Eng. Load [%] : Outport  Port=6  VectorParamsAs1DForOutWhenUnconnected=off
  wires:
  Selector/1 -> x-Thrust L [N]/1
  IO 360 Model/5(Thrust [N]) -> Selector/1, 3D Thrust L [N]/1
  IO 360 Model/19(M_ENG[Nm]) -> 3D Eng. Moment L [Nm]/1
  IO 360 Model/2(RPM) -> Prop. RPM/1
  IO 360 Model/1(MAP[in.Hg]) -> Terminator/1
  IO 360 Model/3(Eng. Pow[W]) -> Terminator1/1
  IO 360 Model/4(Prop. Pow[W]) -> Terminator2/1
  IO 360 Model/6(Prop Pitch [Deg]) -> Terminator3/1
  IO 360 Model/7(FC [gal/h]) -> Fuel flow [gph]/1
  IO 360 Model/8(opt. mix fuel) -> Terminator5/1
  IO 360 Model/9(opt. mix pow) -> Terminator6/1
  IO 360 Model/10(CHT[F]) -> Terminator7/1
  IO 360 Model/11(EGT[F]) -> Terminator8/1
  IO 360 Model/12(Run Con OK?) -> Terminator9/1
  IO 360 Model/13(Limit Gas Rich) -> Terminator10/1
  IO 360 Model/14(Limit Gas Lean) -> Terminator11/1
  IO 360 Model/15(EGT Peak[F]) -> Terminator12/1
  IO 360 Model/16(CHT Peak[F]) -> Terminator4/1
  IO 360 Model/17(OT [F]) -> Terminator13/1
  IO 360 Model/18(OP [psi]) -> Terminator14/1
  IO 360 Model/20(Eng. Load [%]) -> Eng. Load [%]/1
  Throttle  [0...1]/1 -> IO 360 Model/5(Pow. Lever [0...1])
  TAS [m/s]/1 -> IO 360 Model/8(TAS[m/s])
  Prop. Lever [0...1]/1 -> IO 360 Model/6(Prop. Lever [0...1])
  "Mix. Level "/1 -> IO 360 Model/7(Mix. Lever [0...1])
  alpha [rad]/1 -> IO 360 Model/9("AOA [rad] ")
  "Mixture 0: manual 1: opt. pow 2: opt. fuel "/1 -> IO 360 Model/11(Mix option)
  yaw rate/1 -> IO 360 Model/10(yaw rate [rps])
  Rates [rad/s]/1 -> yaw rate/1
  RPM NO/1 -> Set RPM/2
  RPM YES/1 -> Set RPM/1
  set RPM 750<=set RPM<= 2700/1 -> IO 360 Model/12(set RPM)
  Set RPM/1 -> IO 360 Model/13(Activate RPM)
  Altitude [m]/1 -> IO 360 Model/1(H[m])
  Static Pressure [Pa]/1 -> IO 360 Model/2(Pa[N/m^2])
  Air Density [kg/m³]/1 -> IO 360 Model/3(rho[kg/m^3])
  Ait Temperature [K]/1 -> IO 360 Model/4(T [K])

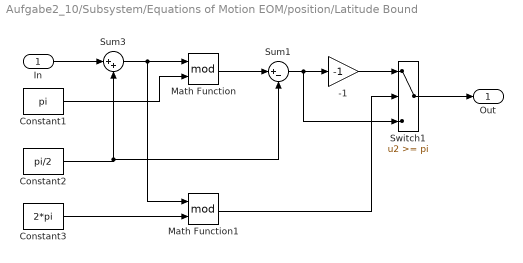
== system Aufgabe2_10/Subsystem/Equations of Motion EOM/position/Latitude Bound ==
  In : Inport
  -1 : Gain  Gain=-1  SaturateOnIntegerOverflow=on  OutDataTypeStr=Inherit: Same as input  ParamDataTypeStr=Inherit: Same as input
  Constant1 : Constant  Value=pi
  Constant2 : Constant  Value=pi/2
  Constant3 : Constant  Value=2*pi
  Math Function : Math  Operator=mod  SignedPower=on
  Math Function1 : Math  Operator=mod  SignedPower=on
  Sum1 : Sum  Inputs=|+-
  Sum3 : Sum  Inputs=|++
  Switch1 : Switch  Threshold=pi  SaturateOnIntegerOverflow=off  InputSameDT=off
  Out : Outport  VectorParamsAs1DForOutWhenUnconnected=off
  wires:
  -1/1 -> Switch1/1
  Switch1/1 -> Out/1
  Math Function/1 -> Sum1/1
  Sum1/1 -> Switch1/3, -1/1
  Constant3/1 -> Math Function1/2
  Constant2/1 -> Sum1/2, Sum3/2
  Constant1/1 -> Math Function/2
  In/1 -> Sum3/1
  Math Function1/1 -> Switch1/2
  Sum3/1 -> Math Function1/1, Math Function/1

== system Aufgabe2_10/Subsystem/Equations of Motion EOM/position/Longitude Bound ==
  In : Inport
  Constant1 : Constant  Value=pi
  Constant3 : Constant  Value=2*pi
  Math Function : Math  Operator=mod  SignedPower=on
  Sum1 : Sum  Inputs=|+-
  Sum3 : Sum  Inputs=|++
  Out : Outport  VectorParamsAs1DForOutWhenUnconnected=off
  wires:
  Sum3/1 -> Math Function/1
  In/1 -> Sum3/1
  Constant1/1 -> Sum1/2, Sum3/2
  Constant3/1 -> Math Function/2
  Math Function/1 -> Sum1/1
  Sum1/1 -> Out/1

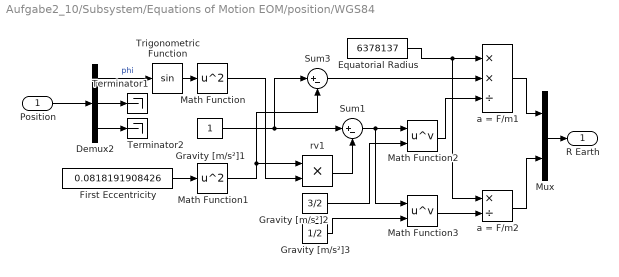
== system Aufgabe2_10/Subsystem/Equations of Motion EOM/position/WGS84 ==
  Position : Inport
  Demux2 : Demux  Outputs=3
  Equatorial Radius : Constant  Value=6378137
  First Eccentricity : Constant  Value=0.0818191908426
  Gravity [m/s²]1 : Constant
  Gravity [m/s²]2 : Constant  Value=3/2
  Gravity [m/s²]3 : Constant  Value=1/2
  Math Function : Math  Operator=square  SignedPower=on
  Math Function1 : Math  Operator=square  SignedPower=on
  Math Function2 : Math  Operator=pow  SignedPower=on
  Math Function3 : Math  Operator=pow  SignedPower=on
  Mux : Mux  Inputs=2
  Sum1 : Sum  Inputs=|+-
  Sum3 : Sum  Inputs=|+-
  Terminator1 : Terminator
  Terminator2 : Terminator
  Trigonometric Function : Trigonometry
  a = F/m1 : Product  Inputs=**/
  a = F/m2 : Product  Inputs=*/
  rv1 : Product
  R Earth : Outport  VectorParamsAs1DForOutWhenUnconnected=off
  wires:
  Gravity [m/s²]2/1 -> Math Function2/2
  a = F/m2/1 -> Mux/2
  Gravity [m/s²]3/1 -> Math Function3/2
  Math Function3/1 -> a = F/m2/2
  First Eccentricity/1 -> Math Function1/1
  Math Function1/1 -> Sum3/2, rv1/1
  Trigonometric Function/1 -> Math Function/1
  rv1/1 -> Sum1/2
  Sum1/1 -> Math Function3/1, Math Function2/1
  Position/1 -> Demux2/1
  Demux2/1 -> Trigonometric Function/1  "phi"
  Demux2/3 -> Terminator2/1
  Demux2/2 -> Terminator1/1
  a = F/m1/1 -> Mux/1
  Math Function/1 -> rv1/2
  Math Function2/1 -> a = F/m1/3
  Equatorial Radius/1 -> a = F/m2/1, a = F/m1/1
  Sum3/1 -> a = F/m1/2
  Gravity [m/s²]1/1 -> Sum1/1, Sum3/1
  Mux/1 -> R Earth/1

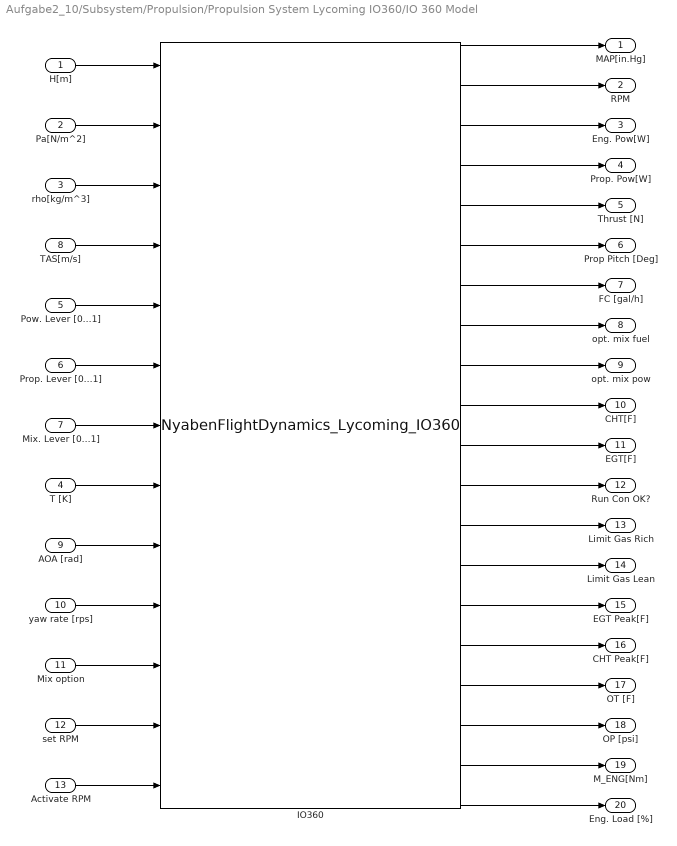
== system Aufgabe2_10/Subsystem/Propulsion/Propulsion System Lycoming IO360/IO 360 Model ==
  H[m] : Inport
  Pa[N/m^2] : Inport  Port=2
  rho[kg/m^3] : Inport  Port=3
  T [K] : Inport  Port=4
  Pow. Lever [0...1] : Inport  Port=5
  Prop. Lever [0...1] : Inport  Port=6
  Mix. Lever [0...1] : Inport  Port=7
  TAS[m/s] : Inport  Port=8
  "AOA [rad] " : Inport  Port=9
  yaw rate [rps] : Inport  Port=10
  Mix option : Inport  Port=11
  set RPM : Inport  Port=12
  Activate RPM : Inport  Port=13
  IO360 : S-Function  FunctionName=NyabenFlightDynamics_Lycoming_IO360  Parameters=Y_TW  SFunctionDeploymentMode=off  EnableBusSupport=off
  MAP[in.Hg] : Outport  VectorParamsAs1DForOutWhenUnconnected=off
  RPM : Outport  Port=2  VectorParamsAs1DForOutWhenUnconnected=off
  Eng. Pow[W] : Outport  Port=3  VectorParamsAs1DForOutWhenUnconnected=off
  Prop. Pow[W] : Outport  Port=4  VectorParamsAs1DForOutWhenUnconnected=off
  Thrust [N] : Outport  Port=5  VectorParamsAs1DForOutWhenUnconnected=off
  Prop Pitch [Deg] : Outport  Port=6  VectorParamsAs1DForOutWhenUnconnected=off
  FC [gal/h] : Outport  Port=7  VectorParamsAs1DForOutWhenUnconnected=off
  opt. mix fuel : Outport  Port=8  VectorParamsAs1DForOutWhenUnconnected=off
  opt. mix pow : Outport  Port=9  VectorParamsAs1DForOutWhenUnconnected=off
  CHT[F] : Outport  Port=10  VectorParamsAs1DForOutWhenUnconnected=off
  EGT[F] : Outport  Port=11  VectorParamsAs1DForOutWhenUnconnected=off
  Run Con OK? : Outport  Port=12  VectorParamsAs1DForOutWhenUnconnected=off
  Limit Gas Rich : Outport  Port=13  VectorParamsAs1DForOutWhenUnconnected=off
  Limit Gas Lean : Outport  Port=14  VectorParamsAs1DForOutWhenUnconnected=off
  EGT Peak[F] : Outport  Port=15  VectorParamsAs1DForOutWhenUnconnected=off
  CHT Peak[F] : Outport  Port=16  VectorParamsAs1DForOutWhenUnconnected=off
  OT [F] : Outport  Port=17  VectorParamsAs1DForOutWhenUnconnected=off
  OP [psi] : Outport  Port=18  VectorParamsAs1DForOutWhenUnconnected=off
  M_ENG[Nm] : Outport  Port=19  VectorParamsAs1DForOutWhenUnconnected=off
  Eng. Load [%] : Outport  Port=20  VectorParamsAs1DForOutWhenUnconnected=off
  wires:
  T [K]/1 -> IO360/8
  Mix. Lever [0...1]/1 -> IO360/7
  Prop. Lever [0...1]/1 -> IO360/6
  Pow. Lever [0...1]/1 -> IO360/5
  TAS[m/s]/1 -> IO360/4
  rho[kg/m^3]/1 -> IO360/3
  Pa[N/m^2]/1 -> IO360/2
  H[m]/1 -> IO360/1
  IO360/1 -> MAP[in.Hg]/1
  IO360/2 -> RPM/1
  IO360/3 -> Eng. Pow[W]/1
  IO360/4 -> Prop. Pow[W]/1
  IO360/5 -> Thrust [N]/1
  IO360/6 -> Prop Pitch [Deg]/1
  IO360/7 -> FC [gal/h]/1
  IO360/8 -> opt. mix fuel/1
  IO360/9 -> opt. mix pow/1
  IO360/10 -> CHT[F]/1
  IO360/11 -> EGT[F]/1
  IO360/12 -> Run Con OK?/1
  IO360/13 -> Limit Gas Rich/1
  IO360/14 -> Limit Gas Lean/1
  IO360/15 -> EGT Peak[F]/1
  IO360/16 -> CHT Peak[F]/1
  IO360/17 -> OT [F]/1
  IO360/18 -> OP [psi]/1
  IO360/19 -> M_ENG[Nm]/1
  yaw rate [rps]/1 -> IO360/10
  "AOA [rad] "/1 -> IO360/9
  Mix option/1 -> IO360/11
  set RPM/1 -> IO360/12
  Activate RPM/1 -> IO360/13
  IO360/20 -> Eng. Load [%]/1
